simulink model "P7_genPlant_RS_NP"  (R2024b)
settings: Solver=VariableStepAuto  StartTime=0.0  StopTime=10.0  RelTol=1e-3
values from neighbouring files (symbols this model uses):
  Ga = 0.112    [P7.m]
  Gf = 1/(Gs*Kd)    (= 0.25)    [P7.m]
  Gs = 0.5    [P7.m]
libraries: cstblocks x3
settings Model: Creator=lucap  LastModifiedBy=lucap

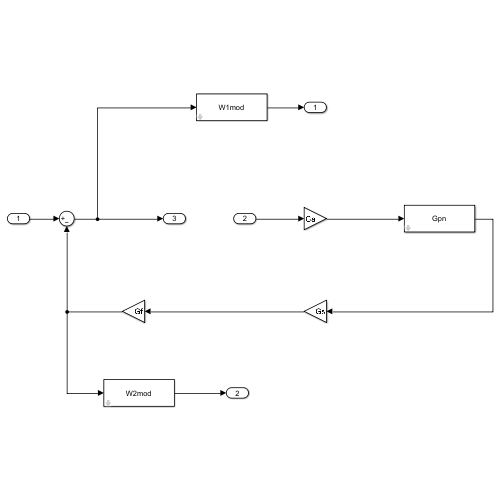
[thumbnail: Simulink's stored preview of the top-level diagram]
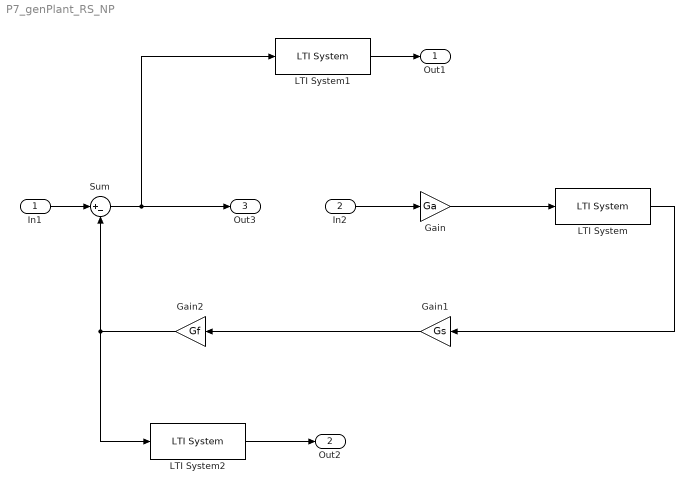
== system P7_genPlant_RS_NP ==
  In1 : Inport
  In2 : Inport  Port=2
  Gain : Gain  Gain=Ga
  Gain1 : Gain  Gain=Gs
  Gain2 : Gain  Gain=Gf
  LTI System : cstblocks/LTI System  sys=Gpn  IC=[]  PadeOrder=0
  LTI System1 : cstblocks/LTI System  sys=W1mod  IC=[]  PadeOrder=0
  LTI System2 : cstblocks/LTI System  sys=W2mod  IC=[]  PadeOrder=0
  Sum : Sum  Inputs=|+-
  Out1 : Outport
  Out2 : Outport  Port=2
  Out3 : Outport  Port=3
  wires:
  Gain/1 -> LTI System/1
  In1/1 -> Sum/1
  Gain1/1 -> Gain2/1
  Gain2/1 -> Sum/2, LTI System2/1
  LTI System/1 -> Gain1/1
  In2/1 -> Gain/1
  Sum/1 -> LTI System1/1, Out3/1
  LTI System2/1 -> Out2/1
  LTI System1/1 -> Out1/1
